simulink model "H8_6GDL_nolineal"  (R2022b)
settings: Solver=VariableStepAuto  StartTime=0.0  StopTime=3  RelTol=1e-3
InitFcn:
  | m = 200;
  | g = 9.81;
  | 
  | x_lev12 = 0.443;
  | x_lev34 = 0.542;
  | x_guid12 = 0.4475;
  | x_guid34 = 0.5465;
  | x_lim = 0.0495;
  | 
  | y_lev13 = 0.23686;
  | y_lev24 = 0.23686;
  | y_guid13 = 0.24263;
  | y_guid24 = 0.24263;
  | y_lim = 0.0005;
  | y_brk = 0.21552;
  | 
  | z_lev = 0.08546;
  | z_guid = 0.026;
  | z_lim = 0.1055;
  | z_brk = 0.03941;
  | 
  | kp_lev = 50;
  | ki_lev = 400;
  | kp_guid = 6;
  | ki_guid = 46.5;
  | 
  | Imax_lev = 50;
  | Imin_lev = -50;
  | Imax_guid = 50;
  | Imin_guid = 0;
  | 
  | cg_nom = 0.567;
  | 
  | I = [43.082 0 0; 0 26.887 -0; 0 0 29.297]
values from neighbouring files (symbols this model uses):
  A5 = argout.a    [linealizacion_5gdl_bien.m]    (also in matrices_linealizacion_5gdl.mat = [0 0 0 0 0 0 0 0 0 0 0 0 ... (100 elements, 10x10)])
  B5 = argout.b    [linealizacion_5gdl_bien.m]    (also in matrices_linealizacion_5gdl.mat = [0 0 0 0 0 -0.000575563603666 -0.0459993641186 -0.0506493386)
  C5 = argout.c    [linealizacion_5gdl_bien.m]    (also in matrices_linealizacion_5gdl.mat = [1 0 0 0 0 0 0 0 0 0 0 1 ... (100 elements, 10x10)])
  cg_suelo = 0.56985    [linealizacion_5gdl_bien.m]    (also in linealizacion_HEMS.m)
  cg_techo = 0.55735    [linealizacion_5gdl_bien.m]    (also in linealizacion_HEMS.m)
  D5 = argout.d    [linealizacion_5gdl_bien.m]    (also in matrices_linealizacion_5gdl.mat = [0 0 0 0 0 0 0 0 0 0 0 0 ... (80 elements, 10x8)])
  Ka = [34.5916764023 4.46928641015 34.7816336405 4.65924364837 92.2484067139 -92.2484067139 74.2332308826 -74.2332308826 -4220.94514487 -4209.6309051 -4205.06787146 -4193.7536317 ... (120 elements, 8x15)]    [Ka.mat]    (also in linealizacion_5gdl_bien.m = place(Aa,Ba,[ -1.5 -1.5 -1.5 -1.5 -2 -2 -6 -6 -7 -7 -5 -5 -2; linealizacion_EMS.m = place(Aa,Ba,[ -1 -1 -2 -2 -3 -3 -6 -6 -7 -7 -5 -5 -4 -4 -5 -)
libraries: slpidlib x16
settings Model: Creator=USUARIO  LastModifiedBy=USUARIO

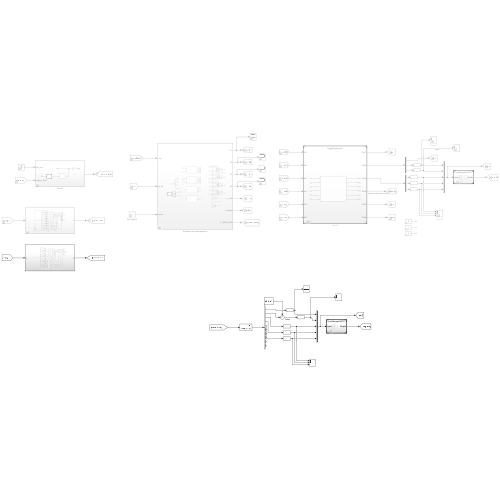
[thumbnail: Simulink's stored preview of the top-level diagram]
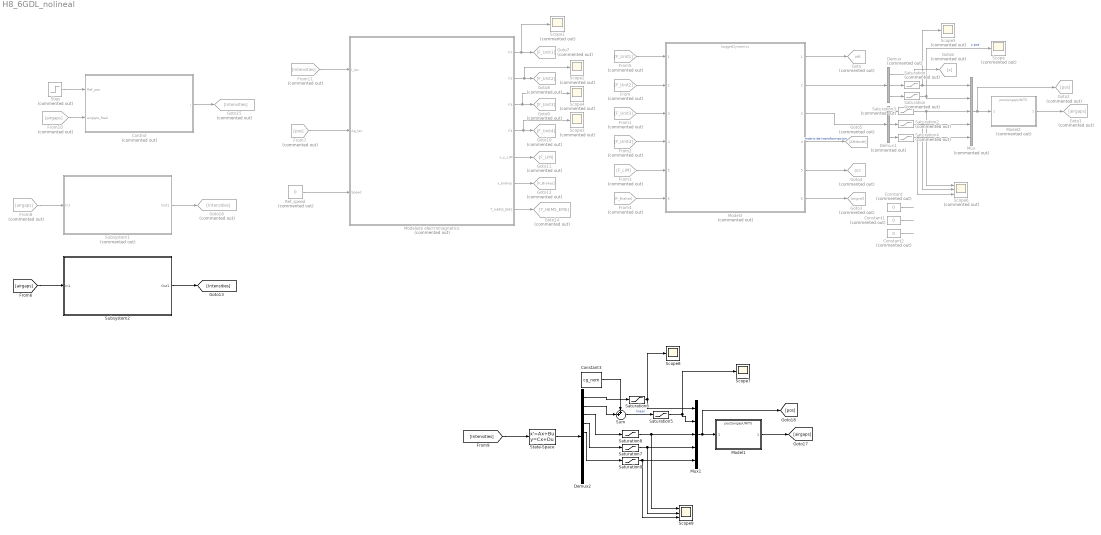
== system H8_6GDL_nolineal ==
  Constant : Constant  Commented=on  Value=0
  Constant1 : Constant  Commented=on  Value=0
  Constant2 : Constant  Commented=on  Value=0
  Constant3 : Constant  Value=cg_nom
  Control : Subsystem  Commented=on
  Demux : Demux  Commented=on  Outputs=3
  Demux1 : Demux  Commented=on  Outputs=3
  Demux2 : Demux  Outputs=10
      settings: DisplayOption=none
  From : From  Commented=on  GotoTag=F_Unit2
  From1 : From  Commented=on  GotoTag=F_Unit3
  From10 : From  Commented=on  GotoTag=airgaps
  From11 : From  Commented=on  GotoTag=Intensities
  From2 : From  Commented=on  GotoTag=F_Unit4
  From3 : From  Commented=on  GotoTag=F_LIM
  From4 : From  Commented=on  GotoTag=F_Brakes
  From5 : From  Commented=on  GotoTag=F_Unit1
  From7 : From  Commented=on  GotoTag=pos
  From8 : From  Commented=on  GotoTag=airgaps
  Goto : Goto  Commented=on  GotoTag=vel  TagVisibility=global
  Goto1 : Goto  Commented=on  GotoTag=airgaps
  Goto10 : Goto  Commented=on  GotoTag=F_Unit4
  Goto11 : Goto  Commented=on  GotoTag=F_LIM
  Goto12 : Goto  Commented=on  GotoTag=F_Brakes
  Goto14 : Goto  Commented=on  GotoTag=T_HEMS_EMS
  Goto15 : Goto  Commented=on  GotoTag=Intensities
  Goto16 : Goto  Commented=on  GotoTag=Intensities
  Goto2 : Goto  Commented=on  GotoTag=pos
  Goto3 : Goto  Commented=on  GotoTag=angvel
  Goto4 : Goto  Commented=on  GotoTag=acc  TagVisibility=global
  Goto5 : Goto  Commented=on  GotoTag=Attitude
  Goto6 : Goto  Commented=on  GotoTag=x
  Goto7 : Goto  Commented=on  GotoTag=F_Unit1
  Goto8 : Goto  Commented=on  GotoTag=F_Unit2
  Goto9 : Goto  Commented=on  GotoTag=F_Unit3
  Model1 : ModelReference  ModelNameDialog=pos2airgapUNITS.slx  SimulationMode=Normal  ModelReferenceVersion=1.3
  Model2 : ModelReference  Commented=on  ModelNameDialog=pos2airgapUNITS.slx  SimulationMode=Normal  ModelReferenceVersion=1.3
  Model3 : ModelReference  Commented=on  ModelNameDialog=boggieDynamics.mdl  SimulationMode=Normal  ModelReferenceVersion=1.21
  Modelado electromagnetico : Subsystem  Commented=on
  Mux : Mux  Commented=on  Inputs=5
  Mux1 : Mux  Inputs=5
  Ref_speed : Constant  Commented=on  Value=0
  Saturation : Saturate  Commented=on  UpperLimit=cg_suelo  LowerLimit=cg_techo
  Saturation1 : Saturate  Commented=on  UpperLimit=0.012  LowerLimit=-0.012
  Saturation2 : Saturate  Commented=on  UpperLimit=0.01268  LowerLimit=-0.01268
  Saturation3 : Saturate  Commented=on  UpperLimit=0.0476  LowerLimit=-0.0476
  Saturation4 : Saturate  Commented=on  UpperLimit=0.024  LowerLimit=-0.024
  Saturation5 : Saturate  UpperLimit=cg_suelo  LowerLimit=cg_techo
  Saturation6 : Saturate  UpperLimit=0.012  LowerLimit=-0.012
  Saturation7 : Saturate  UpperLimit=0.01268  LowerLimit=-0.01268
  Saturation8 : Saturate  UpperLimit=0.0476  LowerLimit=-0.0476
  Saturation9 : Saturate  UpperLimit=0.024  LowerLimit=-0.024
  Scope{,1..5} (6 alike) : Scope  Commented=on
  Scope6 : Scope  Commented=on  NumInputPorts=3
  Scope7 : Scope
  Scope8 : Scope
  Scope9 : Scope  NumInputPorts=3
  State-Space : StateSpace  A=A5  B=B5  C=C5  D=D5  InitialCondition=[-0.001 0.001 0.001 -0.001 0.001 0 0 0 0 0]
  Step : Step  Commented=on  SampleTime=0
  Subsystem1 : Subsystem  Commented=on
  Subsystem2 : Subsystem
  Sum : Sum  Inputs=++|
  wires:
  From2/1 -> Model3/4
  From1/1 -> Model3/3
  From3/1 -> Model3/5
  From/1 -> Model3/2
  From4/1 -> Model3/6
  Model3/4 -> Goto5/1  "matriz de transformacion"
  From5/1 -> Model3/1
  Model3/3 -> Demux1/1
  Mux/1 -> Model2/1, Goto2/1
  Model3/2 -> Demux/1
  Demux/3 -> Saturation/1
  Demux/1 -> Goto6/1
  Model3/1 -> Goto/1
  Demux/2 -> Saturation1/1
  Model3/5 -> Goto4/1
  Model3/6 -> Goto3/1
  Ref_speed/1 -> Modelado electromagnetico/3(Speed)
  From7/1 -> Modelado electromagnetico/2(Ag_lev)
  From11/1 -> Modelado electromagnetico/1(I_lev)
  Modelado electromagnetico/6(x_brakes) -> Goto12/1
  Modelado electromagnetico/5(x_y_LIM) -> Goto11/1
  Modelado electromagnetico/3(F3) -> Scope4/1, Goto9/1
  Modelado electromagnetico/2(F2) -> Scope2/1, Goto8/1
  Modelado electromagnetico/1(F1) -> Scope1/1, Goto7/1
  Modelado electromagnetico/7(T_HEMS_EMS) -> Goto14/1
  From10/1 -> Control/2(airgaps_Real)
  Control/1(I) -> Goto15/1
  Step/1 -> Control/1(Ref_pos)
  Demux1/1 -> Saturation3/1
  Demux1/2 -> Saturation2/1
  Demux1/3 -> Saturation4/1
  Model2/1 -> Goto1/1
  Saturation1/1 -> Scope5/1, Mux/1
  Saturation/1 -> Mux/2, Scope/1  "z pos"
  Saturation3/1 -> Mux/3, Scope6/1
  Saturation2/1 -> Scope6/2, Mux/4
  Saturation4/1 -> Mux/5, Scope6/3
  Modelado electromagnetico/4(F4) -> Scope3/1, Goto10/1
  Subsystem1/1(Out1) -> Goto16/1
  From8/1 -> Subsystem1/1(In1)
  [airgaps] -> Subsystem2/1(In1)
  Subsystem2/1(Out1) -> [Intensities]
  Constant1/1 -> ?
  Constant/1 -> ?
  Constant2/1 -> ?
  [Intensities] -> State-Space/1
  State-Space/1 -> Demux2/1
  Demux2/3 -> Saturation8/1
  Saturation7/1 -> Scope9/2, Mux1/4
  Saturation8/1 -> Mux1/3, Scope9/1
  Demux2/4 -> Saturation7/1
  Saturation9/1 -> Mux1/5, Scope9/3
  Model1/1 -> [airgaps]
  Demux2/5 -> Saturation9/1
  Saturation6/1 -> Mux1/1, Scope8/1
  Demux2/1 -> Saturation6/1
  Mux1/1 -> Model1/1, [pos]
  Constant3/1 -> Sum/1
  Demux2/2 -> Sum/2
  Sum/1 -> Saturation5/1  "lineal"
  Saturation5/1 -> Mux1/2, Scope7/1

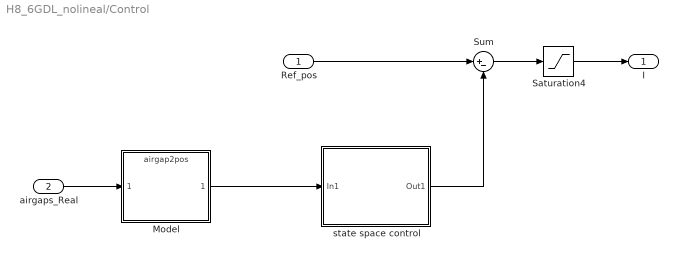
== system H8_6GDL_nolineal/Control ==
  Ref_pos : Inport
  airgaps_Real : Inport  Port=2
  Model : ModelReference  ModelNameDialog=airgap2pos.slx  SimulationMode=Normal  ModelReferenceVersion=1.5
  Saturation4 : Saturate  UpperLimit=55  LowerLimit=-55
  Sum : Sum  Inputs=|+-
  state space control : Subsystem
  I : Outport
  wires:
  airgaps_Real/1 -> Model/1
  Ref_pos/1 -> Sum/1
  Sum/1 -> Saturation4/1
  Saturation4/1 -> I/1
  Model/1 -> state space control/1(In1)
  state space control/1(Out1) -> Sum/2

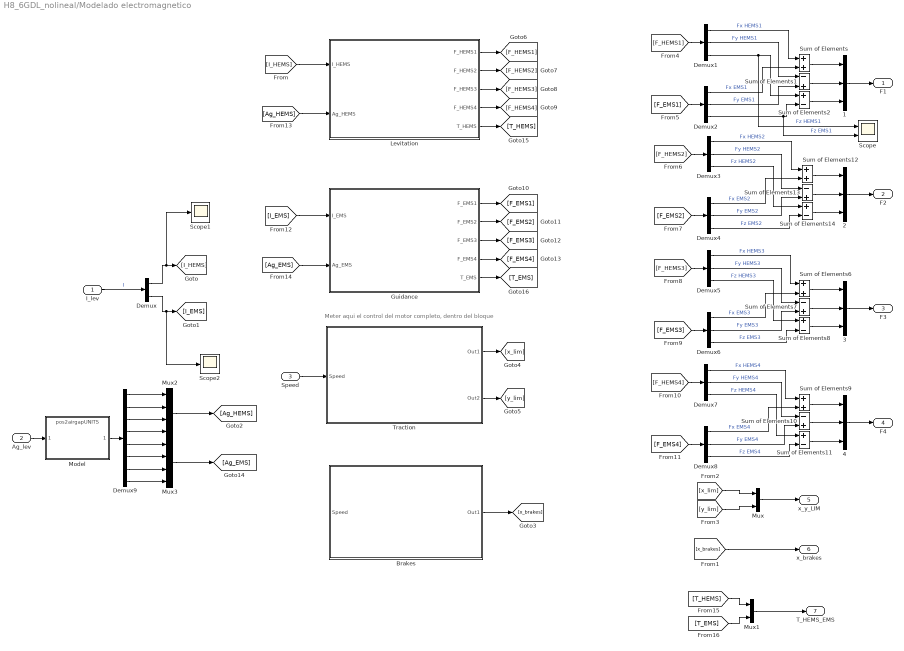
== system H8_6GDL_nolineal/Modelado electromagnetico ==
  note: Meter aqui el control del motor completo, dentro del bloque
  I_lev : Inport
  Ag_lev : Inport  Port=2
  Speed : Inport  Port=3
  {1..4} (4 alike) : Mux  Inputs=3
  Brakes : Subsystem
  Demux : Demux  Outputs=2
  Demux{1..8} (8 alike) : Demux  Outputs=3
  Demux9 : Demux  Outputs=8
  Guidance : Subsystem
  Levitation : Subsystem
  Model : ModelReference  ModelNameDialog=pos2airgapUNITS.slx  SimulationMode=Normal  ModelReferenceVersion=1.3
  Mux : Mux  Inputs=2
  Mux1 : Mux  Inputs=2
  Mux2 : Mux
  Mux3 : Mux
  Scope : Scope  NumInputPorts=2
  Scope1 : Scope
  Scope2 : Scope
  Sum of Elements{,6,9,12} (4 alike) : Sum
  Sum of Elements{1,7,10,13} (4 alike) : Sum  Inputs=-+
  Sum of Elements{2,8,11,14} (4 alike) : Sum  Inputs=+-
  Traction : Subsystem
  F1 : Outport
  F2 : Outport  Port=2
  F3 : Outport  Port=3
  F4 : Outport  Port=4
  x_y_LIM : Outport  Port=5
  x_brakes : Outport  Port=6
  T_HEMS_EMS : Outport  Port=7
  wires:
  I_lev/1 -> Demux/1  "I"
  Demux/1 -> Scope1/1, [I_HEMS]
  Demux/2 -> Scope2/1, [I_EMS]
  [I_HEMS] -> Levitation/1(I_HEMS)
  Brakes/1(Out1) -> [x_brakes]
  [x_brakes] -> x_brakes/1
  Traction/1(Out1) -> [x_lim]
  Traction/2(Out2) -> [y_lim]
  Mux/1 -> x_y_LIM/1
  [x_lim] -> Mux/1
  [y_lim] -> Mux/2
  Levitation/1(F_HEMS1) -> [F_HEMS1]
  Levitation/2(F_HEMS2) -> [F_HEMS2]
  Levitation/3(F_HEMS3) -> [F_HEMS3]
  Levitation/4(F_HEMS4) -> [F_HEMS4]
  Sum of Elements/1 -> 1/1
  1/1 -> F1/1
  Sum of Elements1/1 -> 1/2
  Sum of Elements2/1 -> 1/3
  2/1 -> F2/1
  [F_HEMS1] -> Demux1/1
  Demux1/1 -> Sum of Elements/1  "Fx HEMS1"
  Demux1/2 -> Sum of Elements1/1  "Fy HEMS1"
  Demux1/3 -> Scope/1, Sum of Elements2/1  "Fz HEMS1"
  3/1 -> F3/1
  Sum of Elements8/1 -> 3/3
  Sum of Elements6/1 -> 3/1
  Sum of Elements7/1 -> 3/2
  4/1 -> F4/1
  Sum of Elements11/1 -> 4/3
  Sum of Elements9/1 -> 4/1
  Sum of Elements10/1 -> 4/2
  Guidance/2(F_EMS2) -> [F_EMS2]
  Guidance/3(F_EMS3) -> [F_EMS3]
  Guidance/4(F_EMS4) -> [F_EMS4]
  Guidance/1(F_EMS1) -> [F_EMS1]
  Demux2/1 -> Sum of Elements/2  "Fx EMS1"
  [F_EMS1] -> Demux2/1
  Demux2/2 -> Sum of Elements1/2  "Fy EMS1"
  Demux2/3 -> Scope/2, Sum of Elements2/2  "Fz EMS1"
  [F_EMS2] -> Demux4/1
  Demux4/1 -> Sum of Elements12/2  "Fx EMS2"
  Demux4/2 -> Sum of Elements13/2  "Fy EMS2"
  Sum of Elements14/1 -> 2/3
  Demux3/1 -> Sum of Elements12/1  "Fx HEMS2"
  [F_HEMS2] -> Demux3/1
  Demux3/2 -> Sum of Elements13/1  "Fy HEMS2"
  Demux3/3 -> Sum of Elements14/1  "Fz HEMS2"
  Sum of Elements13/1 -> 2/2
  Sum of Elements12/1 -> 2/1
  Demux4/3 -> Sum of Elements14/2  "Fz EMS2"
  Demux5/3 -> Sum of Elements8/1  "Fz HEMS3"
  Demux5/2 -> Sum of Elements7/1  "Fy HEMS3"
  [F_HEMS3] -> Demux5/1
  Demux6/3 -> Sum of Elements8/2  "Fz EMS3"
  [F_EMS3] -> Demux6/1
  Demux6/1 -> Sum of Elements6/2  "Fx EMS3"
  Demux5/1 -> Sum of Elements6/1  "Fx HEMS3"
  Demux6/2 -> Sum of Elements7/2  "Fy EMS3"
  Demux7/3 -> Sum of Elements11/1  "Fz HEMS4"
  Demux8/3 -> Sum of Elements11/2  "Fz EMS4"
  Demux8/2 -> Sum of Elements10/2  "Fy EMS4"
  Demux7/2 -> Sum of Elements10/1  "Fy HEMS4"
  Demux7/1 -> Sum of Elements9/1  "Fx HEMS4"
  Demux8/1 -> Sum of Elements9/2  "Fx EMS4"
  [F_HEMS4] -> Demux7/1
  [F_EMS4] -> Demux8/1
  [I_EMS] -> Guidance/1(I_EMS)
  Ag_lev/1 -> Model/1
  [Ag_HEMS] -> Levitation/2(Ag_HEMS)
  [Ag_EMS] -> Guidance/2(Ag_EMS)
  Levitation/5(T_HEMS) -> [T_HEMS]
  Speed/1 -> Traction/1(Speed)
  Guidance/5(T_EMS) -> [T_EMS]
  Mux1/1 -> T_HEMS_EMS/1
  [T_HEMS] -> Mux1/1
  [T_EMS] -> Mux1/2
  Model/1 -> Demux9/1
  Demux9/1 -> Mux2/1
  Demux9/2 -> Mux2/2
  Demux9/3 -> Mux2/3
  Demux9/4 -> Mux2/4
  Mux2/1 -> [Ag_HEMS]
  Demux9/5 -> Mux3/1
  Demux9/7 -> Mux3/3
  Mux3/1 -> [Ag_EMS]
  Demux9/6 -> Mux3/2
  Demux9/8 -> Mux3/4

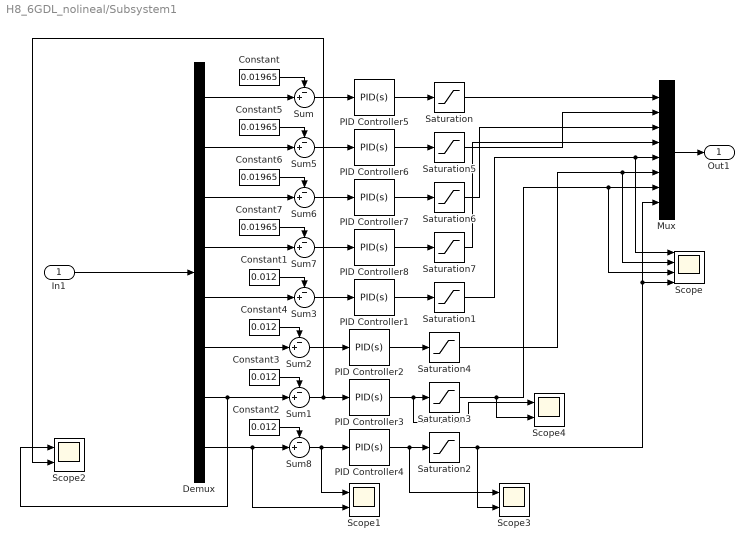
== system H8_6GDL_nolineal/Subsystem1 ==
  In1 : Inport
  Constant{,5..7} (4 alike) : Constant  Value=0.01965
  Constant{1..4} (4 alike) : Constant  Value=0.012
  Demux : Demux  Outputs=8
  Mux : Mux  Inputs=8
  PID Controller{1..4} (4 alike) : slpidlib/PID Controller  Controller=PID  Form=Parallel  TimeDomain=Continuous-time  UseExternalTs=off  SampleTime=-1  IntegratorMethod=Forward Euler  FilterMethod=Forward Euler  ControllerParametersSource=internal  P=6490  I=15500  UseKiTs=off  D=100  N=1900  UseFilter=on  TunerSelectOption=Transfer Function Based (PID Tuner App)  InitialConditionSource=internal  InitialConditionForIntegrator=suelo  InitialConditionForFilter=0  DifferentiatorICPrevScaledInput=0  ExternalReset=none  TrackingMode=off  Kt=1  LimitOutput=off  SatLimitsSource=internal  UpperSaturationLimit=inf  LowerSaturationLimit=-inf  LinearizeAsGain=on  AntiWindupMode=none  Kb=1  LimitIntegrator=off  UpperIntegratorSaturationLimit=inf  LowerIntegratorSaturationLimit=-inf  POutMin=[]  POutMax=[]  IOutMin=[]  IOutMax=[]  DOutMin=[]  DOutMax=[]  NOutMin=[]  NOutMax=[]  SumOutMin=[]  SumOutMax=[]  SaturationOutMin=[]  SaturationOutMax=[]  PParamMin=[]  PParamMax=[]  IParamMin=[]  IParamMax=[]  DParamMin=[]  DParamMax=[]  NParamMin=[]  NParamMax=[]  KbParamMin=[]  KbParamMax=[]  KtParamMin=[]  KtParamMax=[]  KbOutMin=[]  KbOutMax=[]  KtOutMin=[]  KtOutMax=[]  IntegratorOutMin=[]  IntegratorOutMax=[]  FilterOutMin=[]  FilterOutMax=[]  SumI1OutMin=[]  SumI1OutMax=[]  SumI2OutMin=[]  SumI2OutMax=[]  SumI3OutMin=[]  SumI3OutMax=[]  SumI4OutMin=[]  SumI4OutMax=[]  SumDOutMin=[]  SumDOutMax=[]  DifferentiatorOutMin=[]  DifferentiatorOutMax=[]  FilterDiffOutCoefMin=[]  FilterDiffOutCoefMax=[]  ReciprocalOutMin=[]  ReciprocalOutMax=[]  SumDenOutMin=[]  SumDenOutMax=[]  SumNumOutMin=[]  SumNumOutMax=[]  DivideOutMin=[]  DivideOutMax=[]  UdiffTsProdOutMin=[]  UdiffTsProdOutMax=[]  NTsProdOutMin=[]  NTsProdOutMax=[]  UintegralTsProdOutMin=[]  UintegralTsProdOutMax=[]  UngainTsProdOutMin=[]  UngainTsProdOutMax=[]  ClampingZeroOutDataTypeStr=Inherit: Inherit via back propagation  ClampingZeroOutMin=[]  ClampingZeroOutMax=[]  FilterDenConstantOutDataTypeStr=Inherit: Inherit via back propagation  FilterDenConstantOutMin=[]  FilterDenConstantOutMax=[]  PCopyOutDataTypeStr=Inherit: Inherit via back propagation  PCopyOutMin=[]  PCopyOutMax=[]  NCopyOutDataTypeStr=Inherit: Inherit via back propagation  NCopyOutMin=[]  NCopyOutMax=[]  IntegratorContinuousStateAttributes=''  IntegratorStateMustResolveToSignalObject=off  IntegratorRTWStateStorageClass=Auto  FilterContinuousStateAttributes=''  FilterStateMustResolveToSignalObject=off  FilterRTWStateStorageClass=Auto  ParallelPVariant=InternalParameters  IdealPVariant=Disabled  IVariant=InternalParameters  DVariant=InternalParameters  IntegratorVariant=Continuous  SatVariant=Disabled  AWVariant=Passthrough  PCopyVariant=Disabled  TRVariant=Disabled  FdbkBlocksVariant=Forward  IdealPFdbkVariant=Disabled  SatFdbkVariant=Disabled  DerivativeFilterVariant=ContFilter  NVariant=InternalParameters  NCopyVariant=Disabled  FilterICVariant=InternalICsFilter  IntegratorICVariant=InternalICs  ExternalResetVariant=Disabled  TRSumVariant=Passthrough  SumFdbkVariant=Disabled  SumVariant=Sum_PID  TsampFilterVariant=InternalTs  TsampNgainVariant=Passthrough  TsampIntegralVariant=Passthrough  ExternalSaturationOutDataTypeStr=Inherit: Same as second input
  PID Controller{5..8} (4 alike) : slpidlib/PID Controller  Controller=PID  Form=Parallel  TimeDomain=Continuous-time  UseExternalTs=off  SampleTime=-1  IntegratorMethod=Forward Euler  FilterMethod=Forward Euler  ControllerParametersSource=internal  P=64900  I=155000  UseKiTs=off  D=1000  N=1900  UseFilter=on  TunerSelectOption=Transfer Function Based (PID Tuner App)  InitialConditionSource=internal  InitialConditionForIntegrator=suelo  InitialConditionForFilter=0  DifferentiatorICPrevScaledInput=0  ExternalReset=none  TrackingMode=off  Kt=1  LimitOutput=off  SatLimitsSource=internal  UpperSaturationLimit=inf  LowerSaturationLimit=-inf  LinearizeAsGain=on  AntiWindupMode=none  Kb=1  LimitIntegrator=off  UpperIntegratorSaturationLimit=inf  LowerIntegratorSaturationLimit=-inf  POutMin=[]  POutMax=[]  IOutMin=[]  IOutMax=[]  DOutMin=[]  DOutMax=[]  NOutMin=[]  NOutMax=[]  SumOutMin=[]  SumOutMax=[]  SaturationOutMin=[]  SaturationOutMax=[]  PParamMin=[]  PParamMax=[]  IParamMin=[]  IParamMax=[]  DParamMin=[]  DParamMax=[]  NParamMin=[]  NParamMax=[]  KbParamMin=[]  KbParamMax=[]  KtParamMin=[]  KtParamMax=[]  KbOutMin=[]  KbOutMax=[]  KtOutMin=[]  KtOutMax=[]  IntegratorOutMin=[]  IntegratorOutMax=[]  FilterOutMin=[]  FilterOutMax=[]  SumI1OutMin=[]  SumI1OutMax=[]  SumI2OutMin=[]  SumI2OutMax=[]  SumI3OutMin=[]  SumI3OutMax=[]  SumI4OutMin=[]  SumI4OutMax=[]  SumDOutMin=[]  SumDOutMax=[]  DifferentiatorOutMin=[]  DifferentiatorOutMax=[]  FilterDiffOutCoefMin=[]  FilterDiffOutCoefMax=[]  ReciprocalOutMin=[]  ReciprocalOutMax=[]  SumDenOutMin=[]  SumDenOutMax=[]  SumNumOutMin=[]  SumNumOutMax=[]  DivideOutMin=[]  DivideOutMax=[]  UdiffTsProdOutMin=[]  UdiffTsProdOutMax=[]  NTsProdOutMin=[]  NTsProdOutMax=[]  UintegralTsProdOutMin=[]  UintegralTsProdOutMax=[]  UngainTsProdOutMin=[]  UngainTsProdOutMax=[]  ClampingZeroOutDataTypeStr=Inherit: Inherit via back propagation  ClampingZeroOutMin=[]  ClampingZeroOutMax=[]  FilterDenConstantOutDataTypeStr=Inherit: Inherit via back propagation  FilterDenConstantOutMin=[]  FilterDenConstantOutMax=[]  PCopyOutDataTypeStr=Inherit: Inherit via back propagation  PCopyOutMin=[]  PCopyOutMax=[]  NCopyOutDataTypeStr=Inherit: Inherit via back propagation  NCopyOutMin=[]  NCopyOutMax=[]  IntegratorContinuousStateAttributes=''  IntegratorStateMustResolveToSignalObject=off  IntegratorRTWStateStorageClass=Auto  FilterContinuousStateAttributes=''  FilterStateMustResolveToSignalObject=off  FilterRTWStateStorageClass=Auto  ParallelPVariant=InternalParameters  IdealPVariant=Disabled  IVariant=InternalParameters  DVariant=InternalParameters  IntegratorVariant=Continuous  SatVariant=Disabled  AWVariant=Passthrough  PCopyVariant=Disabled  TRVariant=Disabled  FdbkBlocksVariant=Forward  IdealPFdbkVariant=Disabled  SatFdbkVariant=Disabled  DerivativeFilterVariant=ContFilter  NVariant=InternalParameters  NCopyVariant=Disabled  FilterICVariant=InternalICsFilter  IntegratorICVariant=InternalICs  ExternalResetVariant=Disabled  TRSumVariant=Passthrough  SumFdbkVariant=Disabled  SumVariant=Sum_PID  TsampFilterVariant=InternalTs  TsampNgainVariant=Passthrough  TsampIntegralVariant=Passthrough  ExternalSaturationOutDataTypeStr=Inherit: Same as second input
  Saturation{,5..7} (4 alike) : Saturate  UpperLimit=50  LowerLimit=-50
  Saturation{1..4} (4 alike) : Saturate  UpperLimit=50  LowerLimit=0
  Scope : Scope  NumInputPorts=4
  Scope{1..4} (4 alike) : Scope  NumInputPorts=2
  Sum{,1..3,5..8} (8 alike) : Sum  Inputs=-+|
  Out1 : Outport
  wires:
  In1/1 -> Demux/1
  Demux/1 -> Sum/2
  Sum/1 -> PID Controller5/1
  Constant/1 -> Sum/1
  PID Controller5/1 -> Saturation/1
  Mux/1 -> Out1/1
  Saturation/1 -> Mux/1
  Saturation1/1 -> Scope/1, Mux/5
  Sum3/1 -> PID Controller1/1
  PID Controller1/1 -> Saturation1/1
  Demux/5 -> Sum3/2
  Constant1/1 -> Sum3/1
  Demux/8 -> Sum8/2, Scope1/2
  PID Controller4/1 -> Scope3/1, Saturation2/1
  Saturation2/1 -> Scope3/2, Scope/4, Mux/8
  Constant2/1 -> Sum8/1
  Demux/7 -> Sum1/2, Scope2/1
  Constant3/1 -> Sum1/1
  PID Controller3/1 -> Scope4/1, Saturation3/1
  Saturation3/1 -> Scope4/2, Scope/3, Mux/7
  Sum1/1 -> PID Controller3/1, Scope2/2
  Demux/6 -> Sum2/2
  Constant4/1 -> Sum2/1
  PID Controller2/1 -> Saturation4/1
  Saturation4/1 -> Scope/2, Mux/6
  Sum2/1 -> PID Controller2/1
  PID Controller6/1 -> Saturation5/1
  Constant5/1 -> Sum5/1
  Demux/2 -> Sum5/2
  Sum5/1 -> PID Controller6/1
  PID Controller7/1 -> Saturation6/1
  Constant6/1 -> Sum6/1
  Saturation6/1 -> Mux/3
  Demux/3 -> Sum6/2
  Sum6/1 -> PID Controller7/1
  Sum7/1 -> PID Controller8/1
  PID Controller8/1 -> Saturation7/1
  Demux/4 -> Sum7/2
  Constant7/1 -> Sum7/1
  Saturation7/1 -> Mux/4
  Saturation5/1 -> Mux/2
  Sum8/1 -> PID Controller4/1, Scope1/1

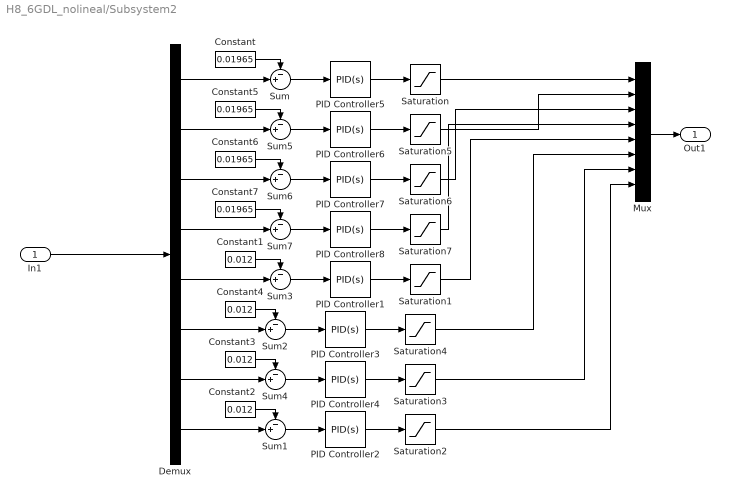
== system H8_6GDL_nolineal/Subsystem2 ==
  In1 : Inport
  Constant{,5..7} (4 alike) : Constant  Value=0.01965
  Constant{1..4} (4 alike) : Constant  Value=0.012
  Demux : Demux  Outputs=8
  Mux : Mux  Inputs=8
  PID Controller{1..4} (4 alike) : slpidlib/PID Controller  Controller=PID  Form=Parallel  TimeDomain=Continuous-time  UseExternalTs=off  SampleTime=-1  IntegratorMethod=Forward Euler  FilterMethod=Forward Euler  ControllerParametersSource=internal  P=5490  I=10500  UseKiTs=off  D=350  N=1900  UseFilter=on  TunerSelectOption=Transfer Function Based (PID Tuner App)  InitialConditionSource=internal  InitialConditionForIntegrator=suelo  InitialConditionForFilter=0  DifferentiatorICPrevScaledInput=0  ExternalReset=none  TrackingMode=off  Kt=1  LimitOutput=off  SatLimitsSource=internal  UpperSaturationLimit=inf  LowerSaturationLimit=-inf  LinearizeAsGain=on  AntiWindupMode=none  Kb=1  LimitIntegrator=off  UpperIntegratorSaturationLimit=inf  LowerIntegratorSaturationLimit=-inf  POutMin=[]  POutMax=[]  IOutMin=[]  IOutMax=[]  DOutMin=[]  DOutMax=[]  NOutMin=[]  NOutMax=[]  SumOutMin=[]  SumOutMax=[]  SaturationOutMin=[]  SaturationOutMax=[]  PParamMin=[]  PParamMax=[]  IParamMin=[]  IParamMax=[]  DParamMin=[]  DParamMax=[]  NParamMin=[]  NParamMax=[]  KbParamMin=[]  KbParamMax=[]  KtParamMin=[]  KtParamMax=[]  KbOutMin=[]  KbOutMax=[]  KtOutMin=[]  KtOutMax=[]  IntegratorOutMin=[]  IntegratorOutMax=[]  FilterOutMin=[]  FilterOutMax=[]  SumI1OutMin=[]  SumI1OutMax=[]  SumI2OutMin=[]  SumI2OutMax=[]  SumI3OutMin=[]  SumI3OutMax=[]  SumI4OutMin=[]  SumI4OutMax=[]  SumDOutMin=[]  SumDOutMax=[]  DifferentiatorOutMin=[]  DifferentiatorOutMax=[]  FilterDiffOutCoefMin=[]  FilterDiffOutCoefMax=[]  ReciprocalOutMin=[]  ReciprocalOutMax=[]  SumDenOutMin=[]  SumDenOutMax=[]  SumNumOutMin=[]  SumNumOutMax=[]  DivideOutMin=[]  DivideOutMax=[]  UdiffTsProdOutMin=[]  UdiffTsProdOutMax=[]  NTsProdOutMin=[]  NTsProdOutMax=[]  UintegralTsProdOutMin=[]  UintegralTsProdOutMax=[]  UngainTsProdOutMin=[]  UngainTsProdOutMax=[]  ClampingZeroOutDataTypeStr=Inherit: Inherit via back propagation  ClampingZeroOutMin=[]  ClampingZeroOutMax=[]  FilterDenConstantOutDataTypeStr=Inherit: Inherit via back propagation  FilterDenConstantOutMin=[]  FilterDenConstantOutMax=[]  PCopyOutDataTypeStr=Inherit: Inherit via back propagation  PCopyOutMin=[]  PCopyOutMax=[]  NCopyOutDataTypeStr=Inherit: Inherit via back propagation  NCopyOutMin=[]  NCopyOutMax=[]  IntegratorContinuousStateAttributes=''  IntegratorStateMustResolveToSignalObject=off  IntegratorRTWStateStorageClass=Auto  FilterContinuousStateAttributes=''  FilterStateMustResolveToSignalObject=off  FilterRTWStateStorageClass=Auto  ParallelPVariant=InternalParameters  IdealPVariant=Disabled  IVariant=InternalParameters  DVariant=InternalParameters  IntegratorVariant=Continuous  SatVariant=Disabled  AWVariant=Passthrough  PCopyVariant=Disabled  TRVariant=Disabled  FdbkBlocksVariant=Forward  IdealPFdbkVariant=Disabled  SatFdbkVariant=Disabled  DerivativeFilterVariant=ContFilter  NVariant=InternalParameters  NCopyVariant=Disabled  FilterICVariant=InternalICsFilter  IntegratorICVariant=InternalICs  ExternalResetVariant=Disabled  TRSumVariant=Passthrough  SumFdbkVariant=Disabled  SumVariant=Sum_PID  TsampFilterVariant=InternalTs  TsampNgainVariant=Passthrough  TsampIntegralVariant=Passthrough  ExternalSaturationOutDataTypeStr=Inherit: Same as second input
  PID Controller{5..8} (4 alike) : slpidlib/PID Controller  Controller=PID  Form=Parallel  TimeDomain=Continuous-time  UseExternalTs=off  SampleTime=-1  IntegratorMethod=Forward Euler  FilterMethod=Forward Euler  ControllerParametersSource=internal  P=64900  I=155000  UseKiTs=off  D=1000  N=1900  UseFilter=on  TunerSelectOption=Transfer Function Based (PID Tuner App)  InitialConditionSource=internal  InitialConditionForIntegrator=suelo  InitialConditionForFilter=0  DifferentiatorICPrevScaledInput=0  ExternalReset=none  TrackingMode=off  Kt=1  LimitOutput=off  SatLimitsSource=internal  UpperSaturationLimit=inf  LowerSaturationLimit=-inf  LinearizeAsGain=on  AntiWindupMode=none  Kb=1  LimitIntegrator=off  UpperIntegratorSaturationLimit=inf  LowerIntegratorSaturationLimit=-inf  POutMin=[]  POutMax=[]  IOutMin=[]  IOutMax=[]  DOutMin=[]  DOutMax=[]  NOutMin=[]  NOutMax=[]  SumOutMin=[]  SumOutMax=[]  SaturationOutMin=[]  SaturationOutMax=[]  PParamMin=[]  PParamMax=[]  IParamMin=[]  IParamMax=[]  DParamMin=[]  DParamMax=[]  NParamMin=[]  NParamMax=[]  KbParamMin=[]  KbParamMax=[]  KtParamMin=[]  KtParamMax=[]  KbOutMin=[]  KbOutMax=[]  KtOutMin=[]  KtOutMax=[]  IntegratorOutMin=[]  IntegratorOutMax=[]  FilterOutMin=[]  FilterOutMax=[]  SumI1OutMin=[]  SumI1OutMax=[]  SumI2OutMin=[]  SumI2OutMax=[]  SumI3OutMin=[]  SumI3OutMax=[]  SumI4OutMin=[]  SumI4OutMax=[]  SumDOutMin=[]  SumDOutMax=[]  DifferentiatorOutMin=[]  DifferentiatorOutMax=[]  FilterDiffOutCoefMin=[]  FilterDiffOutCoefMax=[]  ReciprocalOutMin=[]  ReciprocalOutMax=[]  SumDenOutMin=[]  SumDenOutMax=[]  SumNumOutMin=[]  SumNumOutMax=[]  DivideOutMin=[]  DivideOutMax=[]  UdiffTsProdOutMin=[]  UdiffTsProdOutMax=[]  NTsProdOutMin=[]  NTsProdOutMax=[]  UintegralTsProdOutMin=[]  UintegralTsProdOutMax=[]  UngainTsProdOutMin=[]  UngainTsProdOutMax=[]  ClampingZeroOutDataTypeStr=Inherit: Inherit via back propagation  ClampingZeroOutMin=[]  ClampingZeroOutMax=[]  FilterDenConstantOutDataTypeStr=Inherit: Inherit via back propagation  FilterDenConstantOutMin=[]  FilterDenConstantOutMax=[]  PCopyOutDataTypeStr=Inherit: Inherit via back propagation  PCopyOutMin=[]  PCopyOutMax=[]  NCopyOutDataTypeStr=Inherit: Inherit via back propagation  NCopyOutMin=[]  NCopyOutMax=[]  IntegratorContinuousStateAttributes=''  IntegratorStateMustResolveToSignalObject=off  IntegratorRTWStateStorageClass=Auto  FilterContinuousStateAttributes=''  FilterStateMustResolveToSignalObject=off  FilterRTWStateStorageClass=Auto  ParallelPVariant=InternalParameters  IdealPVariant=Disabled  IVariant=InternalParameters  DVariant=InternalParameters  IntegratorVariant=Continuous  SatVariant=Disabled  AWVariant=Passthrough  PCopyVariant=Disabled  TRVariant=Disabled  FdbkBlocksVariant=Forward  IdealPFdbkVariant=Disabled  SatFdbkVariant=Disabled  DerivativeFilterVariant=ContFilter  NVariant=InternalParameters  NCopyVariant=Disabled  FilterICVariant=InternalICsFilter  IntegratorICVariant=InternalICs  ExternalResetVariant=Disabled  TRSumVariant=Passthrough  SumFdbkVariant=Disabled  SumVariant=Sum_PID  TsampFilterVariant=InternalTs  TsampNgainVariant=Passthrough  TsampIntegralVariant=Passthrough  ExternalSaturationOutDataTypeStr=Inherit: Same as second input
  Saturation{,5..7} (4 alike) : Saturate  UpperLimit=50  LowerLimit=-50
  Saturation{1..4} (4 alike) : Saturate  UpperLimit=50  LowerLimit=0
  Sum{,1..7} (8 alike) : Sum  Inputs=-+|
  Out1 : Outport
  wires:
  In1/1 -> Demux/1
  Demux/1 -> Sum/2
  Sum/1 -> PID Controller5/1
  Constant/1 -> Sum/1
  PID Controller5/1 -> Saturation/1
  Mux/1 -> Out1/1
  Saturation/1 -> Mux/1
  Saturation1/1 -> Mux/5
  Sum3/1 -> PID Controller1/1
  PID Controller1/1 -> Saturation1/1
  Demux/5 -> Sum3/2
  Constant1/1 -> Sum3/1
  Demux/6 -> Sum2/2
  Constant4/1 -> Sum2/1
  PID Controller3/1 -> Saturation4/1
  Saturation4/1 -> Mux/6
  Sum2/1 -> PID Controller3/1
  PID Controller6/1 -> Saturation5/1
  Constant5/1 -> Sum5/1
  Demux/2 -> Sum5/2
  Sum5/1 -> PID Controller6/1
  PID Controller7/1 -> Saturation6/1
  Constant6/1 -> Sum6/1
  Saturation6/1 -> Mux/3
  Demux/3 -> Sum6/2
  Sum6/1 -> PID Controller7/1
  Sum7/1 -> PID Controller8/1
  PID Controller8/1 -> Saturation7/1
  Demux/4 -> Sum7/2
  Constant7/1 -> Sum7/1
  Saturation7/1 -> Mux/4
  Saturation5/1 -> Mux/2
  Sum1/1 -> PID Controller2/1
  Demux/8 -> Sum1/2
  PID Controller2/1 -> Saturation2/1
  Constant2/1 -> Sum1/1
  Sum4/1 -> PID Controller4/1
  Demux/7 -> Sum4/2
  PID Controller4/1 -> Saturation3/1
  Constant3/1 -> Sum4/1
  Saturation3/1 -> Mux/7
  Saturation2/1 -> Mux/8

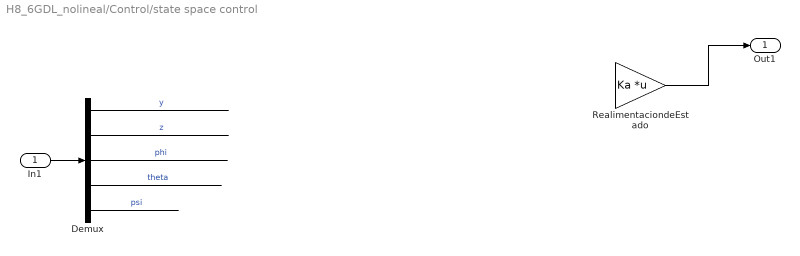
== system H8_6GDL_nolineal/Control/state space control ==
  In1 : Inport
  Demux : Demux  Outputs=5
  RealimentaciondeEstado : Gain  Gain=Ka  Multiplication=Matrix(K*u)
  Out1 : Outport
  wires:
  In1/1 -> Demux/1
  RealimentaciondeEstado/1 -> Out1/1
  Demux/1 -> ?  "y"
  Demux/2 -> ?  "z"
  Demux/3 -> ?  "phi"
  Demux/4 -> ?  "theta"
  Demux/5 -> ?  "psi"

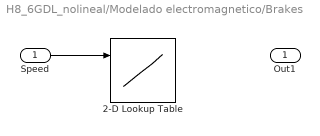
== system H8_6GDL_nolineal/Modelado electromagnetico/Brakes ==
  Speed : Inport
  2-D Lookup Table : Lookup_n-D  BreakpointsForDimension1=[1:3]  BreakpointsForDimension2=[1:3]  InternalRulePriority=Speed  RndMeth=Simplest
      settings: InputPortMap=u0,u1
  Out1 : Outport
  wires:
  Speed/1 -> 2-D Lookup Table/1

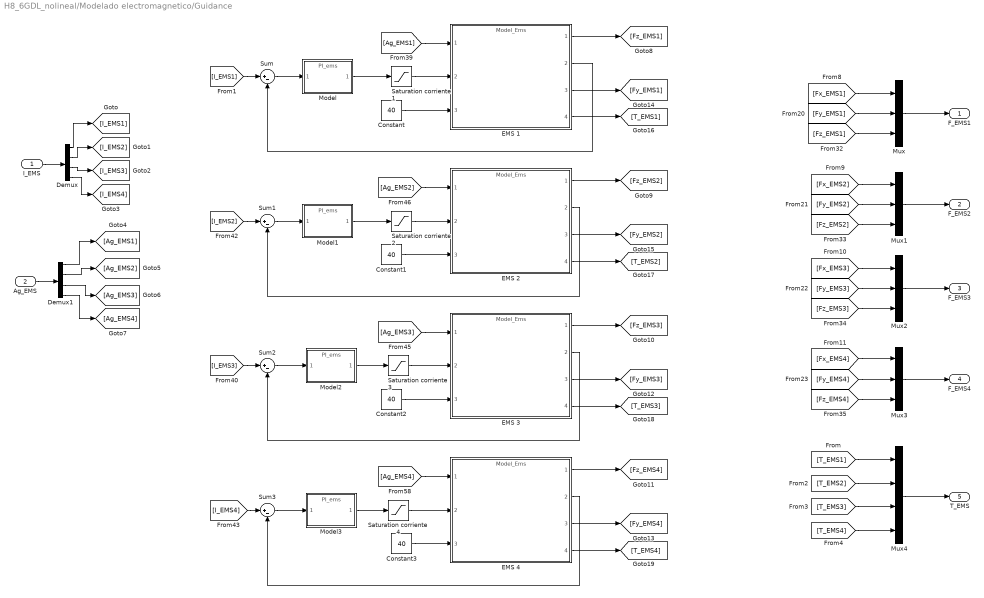
== system H8_6GDL_nolineal/Modelado electromagnetico/Guidance ==
  I_EMS : Inport
  Ag_EMS : Inport  Port=2
  Constant{,1..3} (4 alike) : Constant  Value=40
  Demux : Demux
  Demux1 : Demux
  EMS {1..4} (4 alike) : ModelReference  ModelNameDialog=Model_Ems.slx  SimulationMode=Normal  ModelReferenceVersion=1.21
  Model{,1..3} (4 alike) : ModelReference  ModelNameDialog=PI_ems.slx  SimulationMode=Normal  ModelReferenceVersion=1.2
  Mux{,1..3} (4 alike) : Mux  Inputs=3
  Mux4 : Mux
  Saturation corriente {1..4} (4 alike) : Saturate  UpperLimit=Imax_guid  LowerLimit=Imin_guid
  Sum{,1..3} (4 alike) : Sum  Inputs=|+-
  F_EMS1 : Outport
  F_EMS2 : Outport  Port=2
  F_EMS3 : Outport  Port=3
  F_EMS4 : Outport  Port=4
  T_EMS : Outport  Port=5
  wires:
  [Fz_EMS4] -> Mux3/3
  Demux1/4 -> [Ag_EMS4]
  [Fy_EMS1] -> Mux/2
  I_EMS/1 -> Demux/1
  Mux1/1 -> F_EMS2/1
  Demux/2 -> [I_EMS2]
  [Fy_EMS3] -> Mux2/2
  Mux3/1 -> F_EMS4/1
  [Fy_EMS4] -> Mux3/2
  [Fz_EMS1] -> Mux/3
  Mux/1 -> F_EMS1/1
  Mux2/1 -> F_EMS3/1
  [Fx_EMS3] -> Mux2/1
  Demux1/3 -> [Ag_EMS3]
  Ag_EMS/1 -> Demux1/1
  [Fz_EMS3] -> Mux2/3
  Demux/1 -> [I_EMS1]
  [Fz_EMS2] -> Mux1/3
  [Fx_EMS1] -> Mux/1
  Demux1/1 -> [Ag_EMS1]
  Demux/4 -> [I_EMS4]
  [Fx_EMS2] -> Mux1/1
  [Fy_EMS2] -> Mux1/2
  [Fx_EMS4] -> Mux3/1
  Demux/3 -> [I_EMS3]
  Demux1/2 -> [Ag_EMS2]
  EMS 1/3 -> [Fy_EMS1]
  [Ag_EMS4] -> EMS 4/1
  EMS 4/3 -> [Fy_EMS4]
  EMS 4/1 -> [Fz_EMS4]
  EMS 2/1 -> [Fz_EMS2]
  EMS 1/2 -> Sum/2
  EMS 3/1 -> [Fz_EMS3]
  [Ag_EMS3] -> EMS 3/1
  Constant1/1 -> EMS 2/3
  Constant3/1 -> EMS 4/3
  Constant2/1 -> EMS 3/3
  Constant/1 -> EMS 1/3
  EMS 1/1 -> [Fz_EMS1]
  [Ag_EMS2] -> EMS 2/1
  Model/1 -> Saturation corriente 1/1
  EMS 3/3 -> [Fy_EMS3]
  EMS 2/3 -> [Fy_EMS2]
  [Ag_EMS1] -> EMS 1/1
  Sum/1 -> Model/1
  Sum1/1 -> Model1/1
  EMS 2/2 -> Sum1/2
  [I_EMS2] -> Sum1/1
  Model1/1 -> Saturation corriente 2/1
  [I_EMS1] -> Sum/1
  Sum2/1 -> Model2/1
  EMS 3/2 -> Sum2/2
  [I_EMS3] -> Sum2/1
  Model2/1 -> Saturation corriente 3/1
  Sum3/1 -> Model3/1
  EMS 4/2 -> Sum3/2
  [I_EMS4] -> Sum3/1
  Model3/1 -> Saturation corriente 4/1
  Mux4/1 -> T_EMS/1
  EMS 1/4 -> [T_EMS1]
  EMS 2/4 -> [T_EMS2]
  EMS 3/4 -> [T_EMS3]
  EMS 4/4 -> [T_EMS4]
  [T_EMS1] -> Mux4/1
  [T_EMS2] -> Mux4/2
  [T_EMS3] -> Mux4/3
  [T_EMS4] -> Mux4/4
  Saturation corriente 1/1 -> EMS 1/2
  Saturation corriente 2/1 -> EMS 2/2
  Saturation corriente 3/1 -> EMS 3/2
  Saturation corriente 4/1 -> EMS 4/2

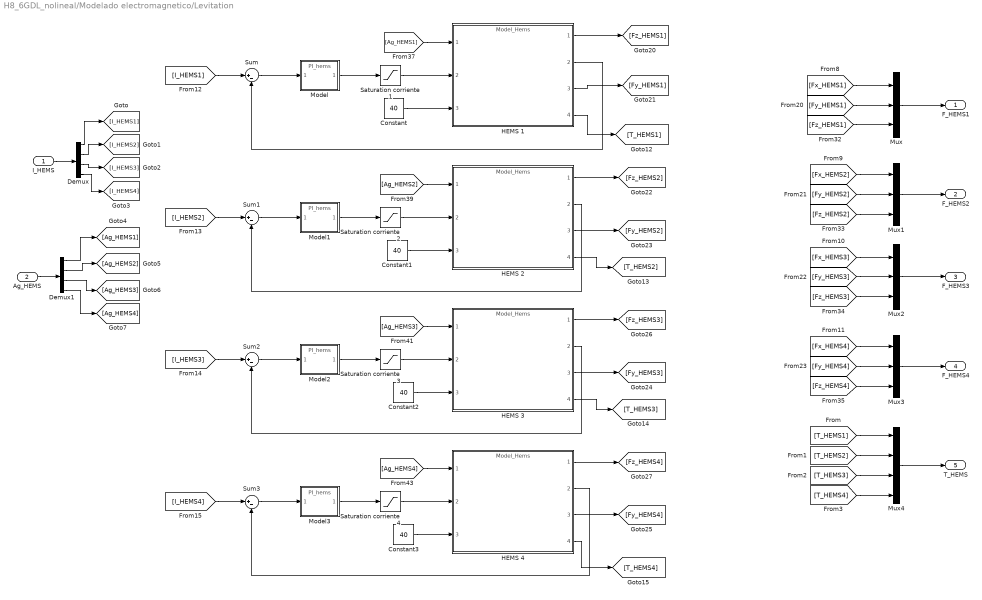
== system H8_6GDL_nolineal/Modelado electromagnetico/Levitation ==
  I_HEMS : Inport
  Ag_HEMS : Inport  Port=2
  Constant{,1..3} (4 alike) : Constant  Value=40
  Demux : Demux
  Demux1 : Demux
  HEMS {1..4} (4 alike) : ModelReference  ModelNameDialog=Model_Hems.slx  SimulationMode=Normal  ModelReferenceVersion=1.18
  Model{,1..3} (4 alike) : ModelReference  ModelNameDialog=PI_hems.slx  SimulationMode=Normal  ModelReferenceVersion=1.3
  Mux{,1..3} (4 alike) : Mux  Inputs=3
  Mux4 : Mux
  Saturation corriente {1..4} (4 alike) : Saturate  UpperLimit=Imax_lev  LowerLimit=Imin_lev
  Sum{,1..3} (4 alike) : Sum  Inputs=|+-
  F_HEMS1 : Outport
  F_HEMS2 : Outport  Port=2
  F_HEMS3 : Outport  Port=3
  F_HEMS4 : Outport  Port=4
  T_HEMS : Outport  Port=5
  wires:
  I_HEMS/1 -> Demux/1
  Mux/1 -> F_HEMS1/1
  Mux1/1 -> F_HEMS2/1
  Mux2/1 -> F_HEMS3/1
  Mux3/1 -> F_HEMS4/1
  Demux/1 -> [I_HEMS1]
  Demux/2 -> [I_HEMS2]
  Demux/3 -> [I_HEMS3]
  Demux/4 -> [I_HEMS4]
  Demux1/2 -> [Ag_HEMS2]
  Demux1/3 -> [Ag_HEMS3]
  Ag_HEMS/1 -> Demux1/1
  Demux1/4 -> [Ag_HEMS4]
  Demux1/1 -> [Ag_HEMS1]
  [Fx_HEMS1] -> Mux/1
  [Fx_HEMS2] -> Mux1/1
  [Fx_HEMS3] -> Mux2/1
  [Fx_HEMS4] -> Mux3/1
  [Fy_HEMS1] -> Mux/2
  [Fy_HEMS2] -> Mux1/2
  [Fy_HEMS3] -> Mux2/2
  [Fy_HEMS4] -> Mux3/2
  [Fz_HEMS1] -> Mux/3
  [Fz_HEMS2] -> Mux1/3
  [Fz_HEMS3] -> Mux2/3
  [Fz_HEMS4] -> Mux3/3
  Model/1 -> Saturation corriente 1/1
  [Ag_HEMS1] -> HEMS 1/1
  HEMS 1/1 -> [Fz_HEMS1]
  HEMS 1/3 -> [Fy_HEMS1]
  HEMS 2/3 -> [Fy_HEMS2]
  HEMS 2/1 -> [Fz_HEMS2]
  [Ag_HEMS2] -> HEMS 2/1
  Model1/1 -> Saturation corriente 2/1
  HEMS 3/3 -> [Fy_HEMS3]
  HEMS 3/1 -> [Fz_HEMS3]
  [Ag_HEMS3] -> HEMS 3/1
  Model2/1 -> Saturation corriente 3/1
  HEMS 4/3 -> [Fy_HEMS4]
  HEMS 4/1 -> [Fz_HEMS4]
  [Ag_HEMS4] -> HEMS 4/1
  Model3/1 -> Saturation corriente 4/1
  Constant1/1 -> HEMS 2/3
  Constant2/1 -> HEMS 3/3
  Constant3/1 -> HEMS 4/3
  HEMS 1/2 -> Sum/2
  Sum/1 -> Model/1
  Sum1/1 -> Model1/1
  HEMS 2/2 -> Sum1/2
  Sum2/1 -> Model2/1
  HEMS 3/2 -> Sum2/2
  Sum3/1 -> Model3/1
  HEMS 4/2 -> Sum3/2
  [I_HEMS1] -> Sum/1
  [I_HEMS2] -> Sum1/1
  [I_HEMS3] -> Sum2/1
  [I_HEMS4] -> Sum3/1
  HEMS 1/4 -> [T_HEMS1]
  Constant/1 -> HEMS 1/3
  HEMS 2/4 -> [T_HEMS2]
  HEMS 3/4 -> [T_HEMS3]
  HEMS 4/4 -> [T_HEMS4]
  Mux4/1 -> T_HEMS/1
  [T_HEMS1] -> Mux4/1
  [T_HEMS4] -> Mux4/4
  [T_HEMS3] -> Mux4/3
  [T_HEMS2] -> Mux4/2
  Saturation corriente 1/1 -> HEMS 1/2
  Saturation corriente 2/1 -> HEMS 2/2
  Saturation corriente 3/1 -> HEMS 3/2
  Saturation corriente 4/1 -> HEMS 4/2

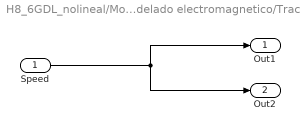
== system H8_6GDL_nolineal/Modelado electromagnetico/Traction ==
  Speed : Inport
  Out1 : Outport
  Out2 : Outport  Port=2
  wires:
  Speed/1 -> Out1/1, Out2/1
